simulink model "mass_spring"  (R2017a)
settings: Solver=FixedStepDiscrete  StartTime=0.0  StopTime=inf  RelTol=1e-3  EnableMultiTasking=on
values from neighbouring files (symbols this model uses):
  PWM_Counter_Period = CPU_frequency/PWM_frequency/2    (= 2250)    [pwmset.m]
undefined symbols (not defined in the file or in its folder): DiscIntNeverNeededParam, Down, GPTRIP1SEL, GPTRIP2SEL, TZ1, TZ2, Up
libraries: c2802xlib x2, c280xlib x2, c2806xlib x2, dspsrcs4 x1, dspsigops x1
settings Model: ExtModeTrigDuration=10  Creator=Kalman  LastModifiedBy=ata.otaran
settings DataIOCC: LimitDataPoints=on  SaveFormat=Array
settings OptimizationCC: LifeSpan=Inf  MaxStackSize=512
settings DebuggingCC: AllowSymbolicDim=off  SFUnexpectedBacktrackingDiag=warning  SFNoUnconditionalDefaultTransitionDiag=warning  SFExecutionAtInitializationDiag=none
settings HardwareCC: ProdBitPerChar=16  ProdBitPerInt=16  ProdBitPerPointer=16  ProdBitPerSizeT=32  ProdBitPerPtrDiffT=32  ProdLargestAtomicInteger=Integer  ProdLargestAtomicFloat=None  ProdWordSize=16  ProdLongLongMode=on  ProdHWDeviceType=Texas Instruments->C2000
settings ModelReferenceCC: PropagateSignalLabelsOutOfModel=off
settings SFSimCC: MATLABDynamicMemAlloc=off
settings RTWCC: SystemTargetFile=ert.tlc  HardwareBoard=TI Piccolo F2806x  TLCOptions=-aInlineSetEventsForThisBaseRateFcn=TLC_FALSE -aSuppressMultiTaskScheduler=TLC_FALSE -aRateBasedStepFcn=1  TemplateMakefile=ert_default_tmf  Description=Embedded Coder  Toolchain=Texas Instruments Code Composer Studio v5 (C2000)
settings CodeAppCC: IgnoreCustomStorageClasses=off
settings ERTTargetCC: CodeReplacementLibrary=TI C28x  MultiwordLength=2048  ConvertIfToSwitch=off  SuppressUnreachableDefaultCases=off
settings ConfigComp: CovMetricSettings=dw  CovHtmlReporting=on  CovSaveCumulativeToWorkspaceVar=on  CovSaveSingleToWorkspaceVar=on  CovExternalEMLEnable=off

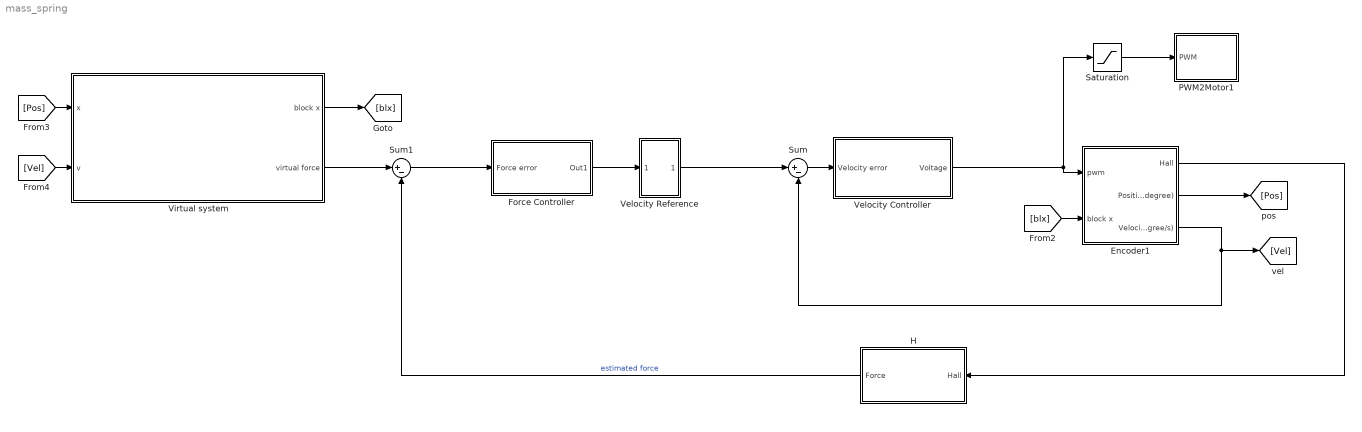
== system mass_spring ==
  Encoder1 : Subsystem
  Force Controller : Subsystem
  H : Subsystem
  PWM2Motor1 : Subsystem
  Saturation : Saturate  UpperLimit=2250  LowerLimit=-2250
  Sum : Sum  Inputs=|+-
  Sum1 : Sum  Inputs=|+-
  Velocity Controller : Subsystem
  Velocity Reference : Subsystem
  Virtual system : Subsystem
  wires:
  Encoder1/2("Position(degree) ") -> [Pos]
  Saturation/1 -> PWM2Motor1/1(PWM)
  Encoder1/3(Velocity(degree/s)) -> Sum/2, [Vel]
  Sum/1 -> Velocity Controller/1("Velocity error ")
  H/1(Force) -> Sum1/2  "estimated force"
  Force Controller/1(Out1) -> Velocity Reference/1(In1)
  Encoder1/1("Hall ") -> H/1(Hall)
  Velocity Reference/1(Out1) -> Sum/1
  Velocity Controller/1(Voltage) -> Saturation/1, Encoder1/1(pwm)
  [blx] -> Encoder1/2(block x)
  Virtual system/1(block x) -> [blx]
  Virtual system/2(virtual force) -> Sum1/1
  Sum1/1 -> Force Controller/1(Force error)
  [Pos] -> Virtual system/1(x)
  [Vel] -> Virtual system/2(v)

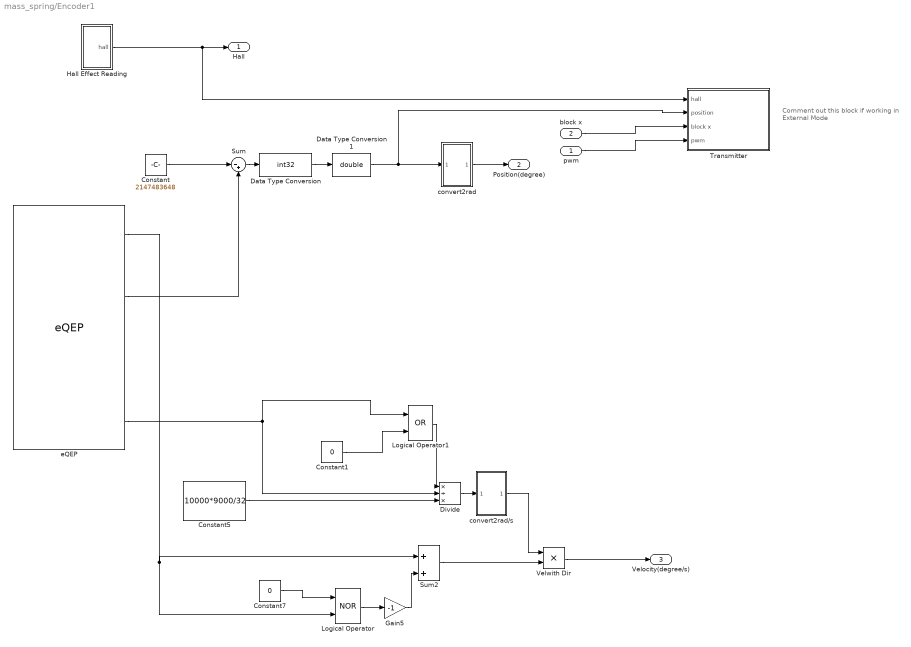
== system mass_spring/Encoder1 ==
  note: Comment out this block if
      | working in External Mode
  pwm : Inport
  block x : Inport  Port=2
  Constant : Constant  Value=2147483648  OutDataTypeStr=uint32
  Constant1 : Constant  Value=0
  Constant5 : Constant  Value=10000*9000/32
  Constant7 : Constant  Value=0
  Data Type Conversion : DataTypeConversion  OutDataTypeStr=int32
  Data Type Conversion1 : DataTypeConversion  OutDataTypeStr=double
  Divide : Product  Inputs=*/*
  Gain5 : Gain  Gain=-1
  Hall Effect Reading : Subsystem
  Logical Operator : Logic  Operator=NOR  AllPortsSameDT=off  OutDataTypeStr=boolean
  Logical Operator1 : Logic  Operator=OR  AllPortsSameDT=off  OutDataTypeStr=boolean
  Sum : Sum  Inputs=|-+
  Sum2 : Sum  Inputs=|++
  Transmitter : Subsystem
  "Velwith Dir " : Product
  convert2rad : Subsystem
  "convert2rad/s " : Subsystem
  eQEP : c280xlib/eQEP  useModule=eQEP1  pcInputmode=Quadrature-count  externalClockrate=2x resolution: Count the rising/falling edge  swapPolarityselection=Clockwise  qdfOutputport=on  qapPolarityselection=off  qbpPolarityselection=off  qipPolarityselection=off  qspPolarityselection=off  igatePolarityselection=off  sampleTime=0.0001  pcOutputport=on  pcMaximumvalue=4294967295  indexInitializationcheck=off  indexInitializationevent=Rising edge  strobeInitializationcheck=off  strobeInitializationevent=Rising edge  softwareInitializationcheck=on  softwareInitializationsource=Set to init value at start up  softwareInitializationmode=on  pcInitialvalue=2147483648  pcResetmode=Reset on an index event  ieloutputport=off  indexEventlatch=Rising edge  seloutputport=off  strobeEventlatch=Rising edge  pcefOutputport=off  enableEqepcapture=on  qctmrOutputport=on  qcprdOutputport=on  captureTimerprescaler=128  upEventprescaler=4  overflowErrorflag=off  directionErrorflag=off  captureTimerposition=On position counter read  unitTimerperiod=1000000000  captureTimerlatch=off  capturePeriodlatch=off  positionCounterlatch=off  soenPolarityselection=off  spselPolarityselection=Index pin is used for sync output  compareValuesource=Specify via dialog  shadowMode=Load on QPOSCNT=0  compareValue=4294967295  syncOutputwidth=1  polaritySyncoutput=Active high  watchdogEnable=off  watchdogTimer=65535  outport1Datatype=auto  outport2Datatype=uint32  outport3Datatype=auto  outport4Datatype=auto  outport5Datatype=auto  outport6Datatype=auto  outport7Datatype=auto  outport8Datatype=auto  outport9Datatype=auto  outport10Datatype=auto  outport11Datatype=auto  outport12Datatype=auto  eqepinterrupt_pce=off  eqepinterrupt_qpe=off  eqepinterrupt_qdc=off  eqepinterrupt_wto=off  eqepinterrupt_pcu=off  eqepinterrupt_pco=off  eqepinterrupt_pcr=off  eqepinterrupt_pcm=off  eqepinterrupt_sel=off  eqepinterrupt_iel=off  eqepinterrupt_uto=off  pheOutputport=off  watchdogOutputport=off  outport13Datatype=auto  outport14Datatype=auto
      settings: SourceProductName=Embedded Coder Support Package for Texas Instruments C2000 Processors  SourceProductBaseCode=TIC2000
  "Hall " : Outport
  "Position(degree) " : Outport  Port=2
  Velocity(degree/s) : Outport  Port=3
  wires:
  "convert2rad/s "/1(Out1) -> "Velwith Dir "/1
  Hall Effect Reading/1(hall) -> Transmitter/1(hall), "Hall "/1
  Logical Operator1/1 -> Divide/1
  Constant5/1 -> Divide/3
  Constant1/1 -> Logical Operator1/2
  Sum2/1 -> "Velwith Dir "/2
  Constant7/1 -> Logical Operator/1
  Logical Operator/1 -> Gain5/1
  Divide/1 -> "convert2rad/s "/1(In1)
  Gain5/1 -> Sum2/2
  eQEP/1 -> Logical Operator/2, Sum2/1
  eQEP/2 -> Sum/2
  Constant/1 -> Sum/1
  eQEP/4 -> Divide/2, Logical Operator1/1
  "Velwith Dir "/1 -> Velocity(degree/s)/1
  Data Type Conversion/1 -> Data Type Conversion1/1
  convert2rad/1(Out1) -> "Position(degree) "/1
  Sum/1 -> Data Type Conversion/1
  Data Type Conversion1/1 -> Transmitter/2(position), convert2rad/1(In1)
  pwm/1 -> Transmitter/4(pwm)
  block x/1 -> Transmitter/3(block x)

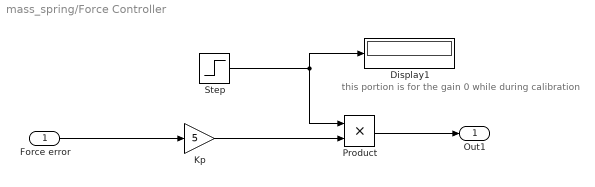
== system mass_spring/Force Controller ==
  note: this portion is for the gain 0 while during calibration
  Force error : Inport
  Display1 : Display
  Kp : Gain  Gain=5
  Product : Product
  Step : Step  Time=0.2
  Out1 : Outport
  wires:
  Force error/1 -> Kp/1
  Product/1 -> Out1/1
  Kp/1 -> Product/2
  Step/1 -> Product/1, Display1/1

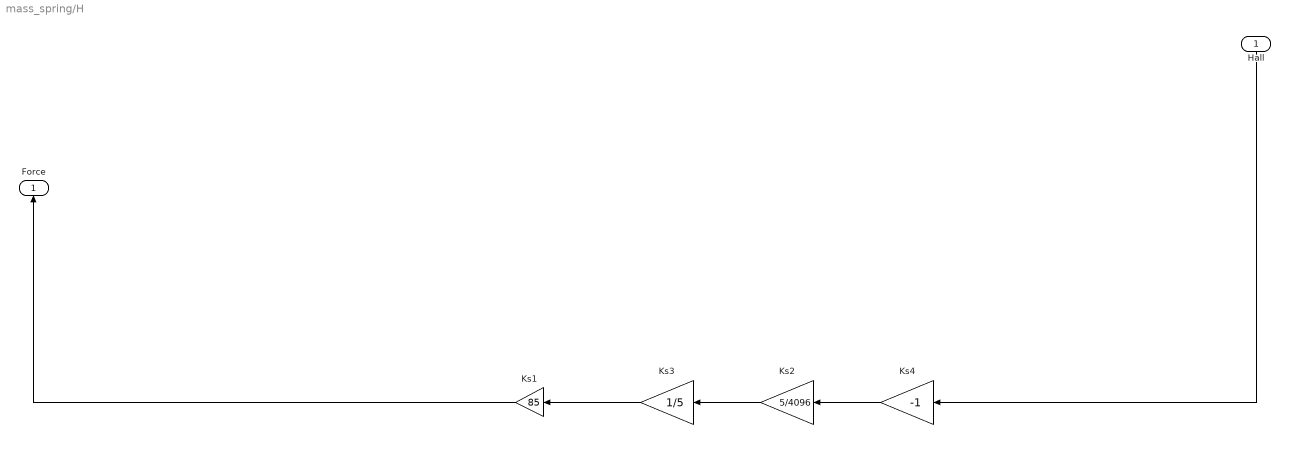
== system mass_spring/H ==
  Hall : Inport
  Ks1 : Gain  Gain=85
  Ks2 : Gain  Gain=5/4096
  Ks3 : Gain  Gain=1/5
  Ks4 : Gain  Gain=-1
  Force : Outport
  wires:
  Hall/1 -> Ks4/1
  Ks1/1 -> Force/1
  Ks4/1 -> Ks2/1
  Ks2/1 -> Ks3/1
  Ks3/1 -> Ks1/1

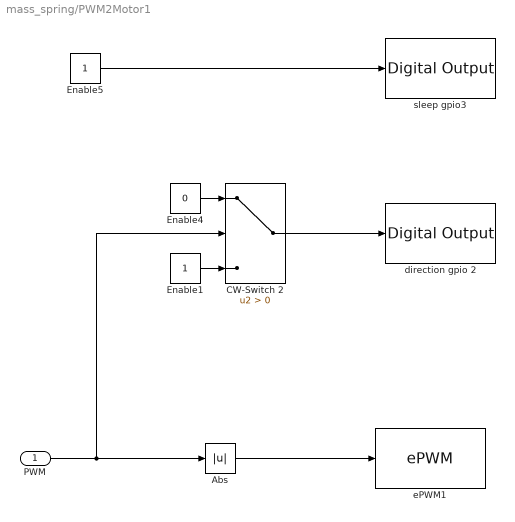
== system mass_spring/PWM2Motor1 ==
  PWM : Inport
  Abs : Abs
  CW-Switch 2 : Switch  Criteria=u2 > Threshold
  Enable1 : Constant
  Enable4 : Constant  Value=0
  Enable5 : Constant
  direction gpio 2 : c2806xlib/Digital Output  GPIO_Number=GPIO0~GPIO7  GPIO_Bit0=off  GPIO_BIT0_Toggle=off  GPIO_Bit1=off  GPIO_BIT1_Toggle=off  GPIO_Bit2=on  GPIO_BIT2_Toggle=off  GPIO_Bit3=off  GPIO_BIT3_Toggle=off  GPIO_Bit4=off  GPIO_BIT4_Toggle=off  GPIO_Bit5=off  GPIO_BIT5_Toggle=off  GPIO_Bit6=off  GPIO_BIT6_Toggle=off  GPIO_Bit7=off  GPIO_BIT7_Toggle=off
      settings: SourceProductName=Embedded Coder Support Package for Texas Instruments C2000 Processors  SourceProductBaseCode=TIC2000
  ePWM1 : c2802xlib/ePWM  useModule=ePWM1  ePWMxLINKTBPRD=Not Linked  periodUnits=Clock cycles  timerSource=Specify via dialog  timerPeriod_clk=PWM_Counter_Period+1  timerPeriod_sec=0.0001  tbshadow=Counter equals to zero  countingMode=Up-Down  phaseActiveEnable=Disable  phaseDirection=Count down after sync  phaseActive=0  synchronizationEnable=off  dcaevt1Sync=off  dcbevt1Sync=off  synchronizationOption=Disable  clockPrescale=1  HSclockPrescale=1  enswap=off  ePWMxAStatus=on  ePWMxAactionLogic1=Do nothing  ePWMxAactionLogic2=Do nothing  ePWMxAactionLogic3=Clear  ePWMxAactionLogic4=Set  ePWMxAactionLogic5=Do nothing  ePWMxAactionLogic6=Do nothing  ePWMxALoadMode=Load on counter equals to zero (CTR=Zero)  ePWMxACSFenable=off  ePWMxACSFvalue=Forcing disable  ePWMxASFreload=Zero  ePWMxBStatus=off  ePWMxBactionLogic1=Set  ePWMxBactionLogic2=Clear  ePWMxBactionLogic3=Do nothing  ePWMxBactionLogic4=Do nothing  ePWMxBactionLogic5=Clear  ePWMxBactionLogic6=Set  ePWMxBLoadMode=Load on counter equals to zero (CTR=Zero)  ePWMxBCSFenable=off  ePWMxBCSFvalue=Forcing disable  ePWMxBSFreload=Zero  ePWNxBOutWay=off  ePWMxLINKCMPA=Not Linked  CMPAUnits=Clock cycles  CMPASource=Input port  CMPAValue_per=50  CMPAValue_clk=PWM_Counter_Period/2+1  enCMPAshadow=Counter equals to zero  ePWMxLINKCMPB=Not Linked  CMPBUnits=Clock cycles  CMPBSource=Specify via dialog  CMPBValue_per=50  CMPBValue_clk=PWM_Counter_Period/2+1  enCMPBshadow=Counter equals to zero  ePWMxLINKCMPC=Not Linked  CMPCUnits=Clock cycles  CMPCSource=Specify via dialog  CMPCValue_per=50  CMPCValue_clk=32000  enCMPCshadow=Counter equals to zero  ePWMxLINKCMPD=Not Linked  CMPDUnits=Clock cycles  CMPDSource=Specify via dialog  CMPDValue_per=50  CMPDValue_clk=32000  enCMPDshadow=Counter equals to zero  enableDBePWMxA=off  enableDBePWMxB=off  enhalfcycle=off  DBpolarity=Active high (AH)  DBedgeDelay=Positive  DBSource_ePWMxA=ePWMxA  DBSource_ePWMxB=ePWMxA  DBperiodSource=Specify via dialog  REDperiod=0  FEDperiod=0  adcstartModuleA=off  adcrequestEventA=First event  adcstartEventA=Digital Compare Module A Event 1 start of conversion (DCAEVT1.soc)  adcstartEventA_type2=Digital Compare Module A Event 1 start of conversion (DCAEVT1.soc)  adcstartModuleB=off  adcrequestEventB=First event  adcstartEventB=Counter equals to zero (CTR=Zero)  adcstartEventB_type2=Counter equals to zero (CTR=Zero)  intEn=off  intPrd=First event  intSel=Counter equals to zero (CTR=Zero)  intSel_type2=Counter equals to zero (CTR=Zero)  hrpe=off  enHRPWM=off  HRPWM_LoadMode=Counter equals to period (CTR=PRD)  HRPWM_CTLMode=Duty or Period control mode  HRPWM_EDGMode=Both edge  hrpeb=off  enHRPWMB=off  HRPWM_LoadModeB=Counter equals to zero (CTR=ZERO)  HRPWM_CTLModeB=Duty or Period control mode  HRPWM_EDGModeB=Both edge  enSFO=on  enautoconv=on  chopperEnable=off  chopperFrequency=1  chopperFirstwidth=1  chopperDuty=12.5%  tripZonesource=Specify via dialog  tzselOSHT1=off  tzselOSHT2=off  tzselOSHT3=off  tzselOSHDCAEV1=off  tzselOSHDCBEV1=off  tzselCBC1=off  tzselCBC2=off  tzselCBC3=off  tzselCBCDCAEV2=off  tzselCBCDCBEV2=off  tzselOSHT4=off  tzselOSHT5=off  tzselOSHT6=off  tzselCBC4=off  tzselCBC5=off  tzselCBC6=off  enTzOstIntr=off  enTzCbcIntr=off  enTzDCAEVT1Intr=off  enTzDCAEVT2Intr=off  enTzDCBEVT1Intr=off  enTzDCBEVT2Intr=off  ePWMxAforced=No action  ePWMxBforced=No action  DCAEVT1forced=No action  DCBEVT1forced=No action  DCAEVT2forced=No action  DCBEVT2forced=No action  dcah=Trip Zone 1 input (TZ1)  dcal=Trip Zone 2 input (TZ2)  dcbh=Trip Zone 1 input (TZ1)  dcbl=Trip Zone 2 input (TZ2)  dcah_type2=GPTRIP1SEL/(TZ1)  dcal_type2=GPTRIP2SEL/(TZ2)  dcbh_type2=GPTRIP1SEL/(TZ1)  dcbl_type2=GPTRIP2SEL/(TZ2)  gendcaevt1=Event disabled  gendcaevt2=Event disabled  gendcbevt1=Event disabled  gendcbevt2=Event disabled  dcaevt1src=DCAEVT1 with sync  dcaevt2src=DCAEVT2 with sync  dcbevt1src=DCBEVT1 with sync  dcbevt2src=DCBEVT2 with sync  pulsesel=Counter equals to zero (CTR=Zero)  blankinv=off  blankoffset=0  blankwidth=0  evsrcsel=Filtered version of DCAEVT1 (DCAEVT1FILT)  encape=off  PwmType=C2000
      settings: SourceProductName=Embedded Coder Support Package for Texas Instruments C2000 Processors
  sleep gpio3 : c2806xlib/Digital Output  GPIO_Number=GPIO0~GPIO7  GPIO_Bit0=off  GPIO_BIT0_Toggle=off  GPIO_Bit1=off  GPIO_BIT1_Toggle=off  GPIO_Bit2=off  GPIO_BIT2_Toggle=off  GPIO_Bit3=on  GPIO_BIT3_Toggle=off  GPIO_Bit4=off  GPIO_BIT4_Toggle=off  GPIO_Bit5=off  GPIO_BIT5_Toggle=off  GPIO_Bit6=off  GPIO_BIT6_Toggle=off  GPIO_Bit7=off  GPIO_BIT7_Toggle=off
      settings: SourceProductName=Embedded Coder Support Package for Texas Instruments C2000 Processors  SourceProductBaseCode=TIC2000
  wires:
  PWM/1 -> Abs/1, CW-Switch 2/2
  Enable1/1 -> CW-Switch 2/3
  Enable4/1 -> CW-Switch 2/1
  Enable5/1 -> sleep gpio3/1
  CW-Switch 2/1 -> direction gpio 2/1
  Abs/1 -> ePWM1/1

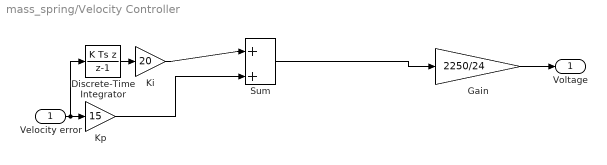
== system mass_spring/Velocity Controller ==
  "Velocity error " : Inport
  Discrete-Time Integrator : DiscreteIntegrator  IntegratorMethod=Integration: Backward Euler  InitialConditionSetting=State (most efficient)  SampleTime=-1  ICPrevOutput=DiscIntNeverNeededParam  ICPrevScaledInput=DiscIntNeverNeededParam
  Gain : Gain  Gain=2250/24
  Ki : Gain  Gain=20
  Kp : Gain  Gain=15
  Sum : Sum  Inputs=|++
  Voltage : Outport
  wires:
  "Velocity error "/1 -> Discrete-Time Integrator/1, Kp/1
  Kp/1 -> Sum/2
  Ki/1 -> Sum/1
  Sum/1 -> Gain/1
  Discrete-Time Integrator/1 -> Ki/1
  Gain/1 -> Voltage/1

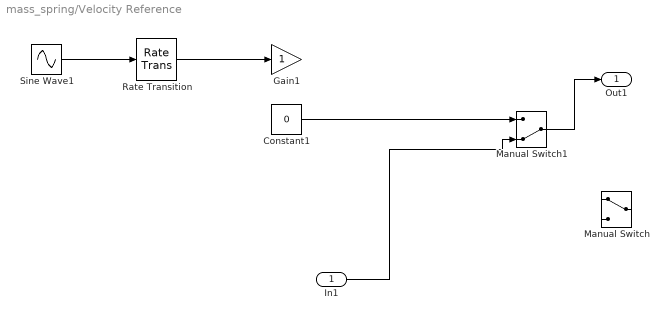
== system mass_spring/Velocity Reference ==
  In1 : Inport
  Constant1 : Constant  Value=0
  Gain1 : Gain
  Manual Switch : ManualSwitch
  Manual Switch1 : ManualSwitch  CurrentSetting=0
  Rate Transition : RateTransition
  Sine Wave1 : Sin  Amplitude=pi  Frequency=2*pi  SampleTime=1e-3
  Out1 : Outport
  wires:
  In1/1 -> Manual Switch1/2
  Rate Transition/1 -> Gain1/1
  Constant1/1 -> Manual Switch1/1
  Sine Wave1/1 -> Rate Transition/1
  Manual Switch1/1 -> Out1/1

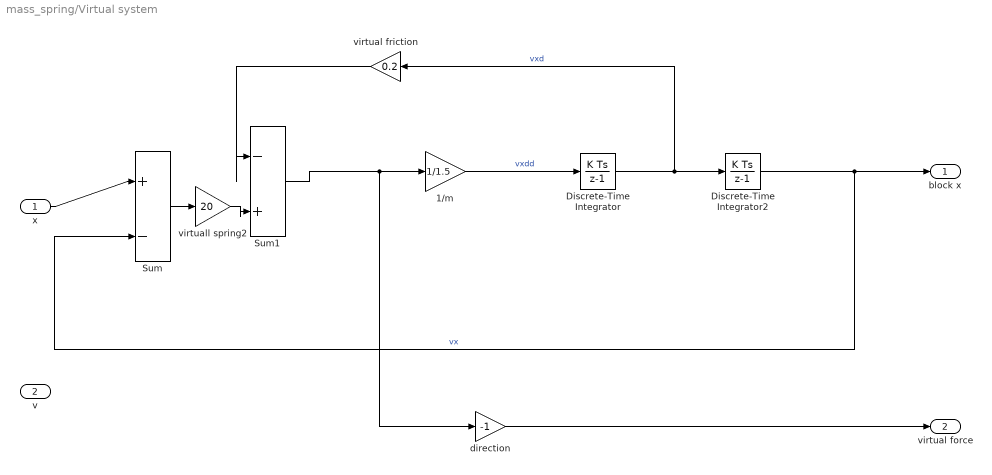
== system mass_spring/Virtual system ==
  x : Inport
  v : Inport  Port=2
  " virtual friction" : Gain  Gain=0.2
  1/m : Gain  Gain=1/1.5
  Discrete-Time Integrator : DiscreteIntegrator  InitialConditionSetting=State (most efficient)  SampleTime=-1  ICPrevOutput=DiscIntNeverNeededParam  ICPrevScaledInput=DiscIntNeverNeededParam
  Discrete-Time Integrator2 : DiscreteIntegrator  InitialConditionSetting=State (most efficient)  SampleTime=-1  ICPrevOutput=DiscIntNeverNeededParam  ICPrevScaledInput=DiscIntNeverNeededParam
  Sum : Sum  Inputs=|+-
  Sum1 : Sum  Inputs=|-+
  direction : Gain  Gain=-1
  virtuall spring2 : Gain  Gain=20
  block x : Outport
  virtual force : Outport  Port=2
  wires:
  Discrete-Time Integrator/1 -> " virtual friction"/1, Discrete-Time Integrator2/1  "vxd"
  Discrete-Time Integrator2/1 -> block x/1, Sum/2  "vx"
  Sum1/1 -> 1/m/1, direction/1
  x/1 -> Sum/1
  1/m/1 -> Discrete-Time Integrator/1  "vxdd"
  Sum/1 -> virtuall spring2/1
  virtuall spring2/1 -> Sum1/2
  " virtual friction"/1 -> Sum1/1
  direction/1 -> virtual force/1

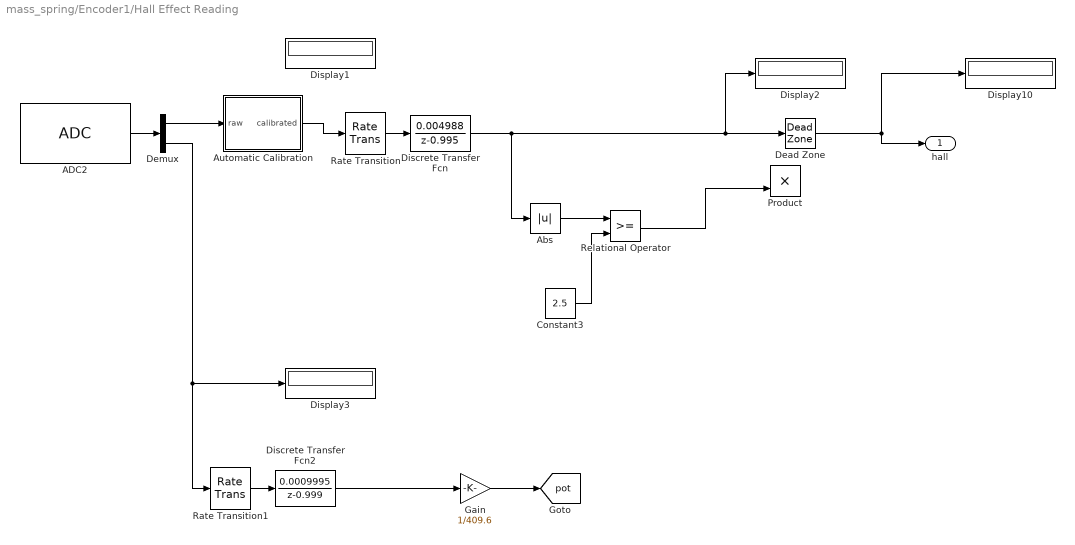
== system mass_spring/Encoder1/Hall Effect Reading ==
  ADC2 : c2802xlib/ADC  ADCModule=1  samplingMode=Simultaneous sample mode  ADCResolution=12-bit (Single-ended input)  useSOC1=SOC1  useSOC2=SOC0_SOC1  SOCAcquisitionWindow=7  SOCTriggerSource=Software  SOCInterruptTrigger=No ADCINT  Ts=-1  dType=int32  postInterrupt=off  interruptSel=ADCINT1  ADCINTContinuous=off  endma=off  chdma=1  blkParamProc=C2000  conv1=ADCINA7  conv2=ADCINA7 and ADCINB7  conv1_Type4=ADCIN0  conv2_Type4=ADCIN0 and ADCIN1
      settings: SourceProductName=Embedded Coder Support Package for Texas Instruments C2000 Processors
  Abs : Abs
  Automatic Calibration : Subsystem
  Constant3 : Constant  Value=2.5
  Dead Zone : DeadZone  LowerValue=-2.5  UpperValue=2.5  SaturateOnIntegerOverflow=on
  Demux : Demux  Outputs=2
  Discrete Transfer Fcn : DiscreteTransferFcn  Numerator=[0.004988]  Denominator=[1 -0.995]
  Discrete Transfer Fcn2 : DiscreteTransferFcn  Numerator=[0.0009995]  Denominator=[1 -0.999]
  Display{1..3,10} (4 alike) : Display
  Gain : Gain  Gain=1/409.6  OutDataTypeStr=double
  Product : Product
  Rate Transition : RateTransition
  Rate Transition1 : RateTransition
  Relational Operator : RelationalOperator  OutDataTypeStr=boolean  RndMeth=Nearest
  hall : Outport
  tag scope: pot=global
  wires:
  Abs/1 -> Relational Operator/1
  Constant3/1 -> Relational Operator/2
  Relational Operator/1 -> Product/2
  Automatic Calibration/1(calibrated) -> Rate Transition/1
  Rate Transition/1 -> Discrete Transfer Fcn/1
  ADC2/1 -> Demux/1
  Demux/2 -> Display3/1, Rate Transition1/1
  Rate Transition1/1 -> Discrete Transfer Fcn2/1
  Discrete Transfer Fcn2/1 -> Gain/1
  Discrete Transfer Fcn/1 -> Abs/1, Dead Zone/1, Display2/1
  Gain/1 -> [pot]
  Dead Zone/1 -> hall/1, Display10/1
  Demux/1 -> Automatic Calibration/1(raw)

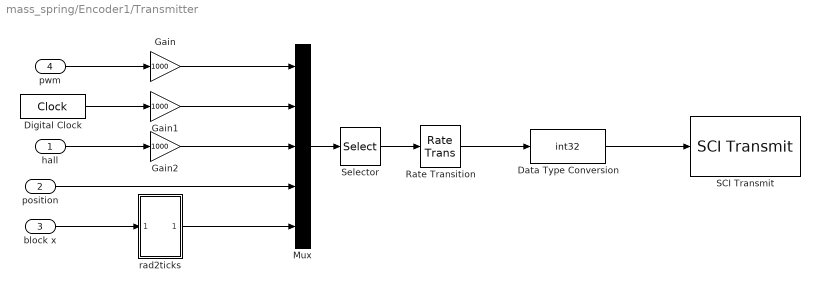
== system mass_spring/Encoder1/Transmitter ==
  hall : Inport
  position : Inport  Port=2
  block x : Inport  Port=3
  pwm : Inport  Port=4
  Data Type Conversion : DataTypeConversion  OutDataTypeStr=int32  ConvertRealWorld=Stored Integer (SI)
  Digital Clock : DigitalClock  SampleTime=0.0001
  Gain : Gain  Gain=1000
  Gain1 : Gain  Gain=1000
  Gain2 : Gain  Gain=1000
  Mux : Mux  Inputs=5
  Rate Transition : RateTransition  Integrity=off  OutPortSampleTime=0.01
  SCI Transmit : c280xlib/SCI Transmit  sciModule=A  dataHead='S'  dataTail='E'  postInterrupt=on  numFifo=3
      settings: SourceProductName=Embedded Coder Support Package for Texas Instruments C2000 Processors
  Selector : Selector  InputPortWidth=5  IndexOptions=Index vector (dialog)  Indices=[4 5]  OutputSizes=1
  rad2ticks : Subsystem
  wires:
  rad2ticks/1(Out1) -> Mux/5
  position/1 -> Mux/4
  Rate Transition/1 -> Data Type Conversion/1
  Data Type Conversion/1 -> SCI Transmit/1
  block x/1 -> rad2ticks/1(In1)
  Digital Clock/1 -> Gain1/1
  Gain/1 -> Mux/1
  pwm/1 -> Gain/1
  hall/1 -> Gain2/1
  Mux/1 -> Selector/1
  Gain1/1 -> Mux/2
  Gain2/1 -> Mux/3
  Selector/1 -> Rate Transition/1

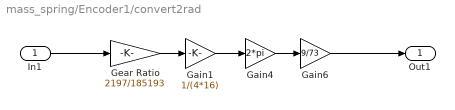
== system mass_spring/Encoder1/convert2rad ==
  In1 : Inport
  Gain1 : Gain  Gain=1/(4*16)
  Gain4 : Gain  Gain=2*pi
  Gain6 : Gain  Gain=9/73
  Gear Ratio : Gain  Gain=2197/185193
  Out1 : Outport
  wires:
  Gain1/1 -> Gain4/1
  Gear Ratio/1 -> Gain1/1
  Gain4/1 -> Gain6/1
  In1/1 -> Gear Ratio/1
  Gain6/1 -> Out1/1

== system mass_spring/Encoder1/convert2rad//s  ==
  In1 : Inport
  Gain1 : Gain  Gain=1/(4*16)
  Gain4 : Gain  Gain=2*pi
  Gain6 : Gain  Gain=9/73
  Gear Ratio : Gain  Gain=2197/185193
  Out1 : Outport
  wires:
  Gain6/1 -> Out1/1
  In1/1 -> Gear Ratio/1
  Gain4/1 -> Gain6/1
  Gear Ratio/1 -> Gain1/1
  Gain1/1 -> Gain4/1

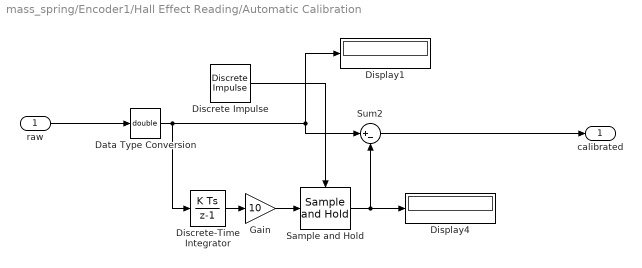
== system mass_spring/Encoder1/Hall Effect Reading/Automatic Calibration ==
  raw : Inport
  Data Type Conversion : DataTypeConversion  OutDataTypeStr=double
  Discrete Impulse : dspsrcs4/Discrete  Impulse  Delay=1000  SampleTime=-1  FrameSample=1  OutputFrames=off  dataType=double  isSigned=on  wordLen=16  udDataType=sfix(16)  fracBitsMode=Best precision  numFracBits=15  OutDataTypeStr=double  LastOutDataTypeStr=double
  Discrete-Time Integrator : DiscreteIntegrator  InitialConditionSetting=State (most efficient)  SampleTime=0.0001  ICPrevOutput=DiscIntNeverNeededParam  ICPrevScaledInput=DiscIntNeverNeededParam
  Display1 : Display
  Display4 : Display
  Gain : Gain  Gain=10
  Sample and Hold : dspsigops/Sample and Hold  trig=Rising edge  initCond=0  latchinput=off
  Sum2 : Sum  Inputs=|+-
  calibrated : Outport
  wires:
  raw/1 -> Data Type Conversion/1
  Discrete Impulse/1 -> Sample and Hold/Trigger
  Data Type Conversion/1 -> Discrete-Time Integrator/1, Sum2/1, Display1/1
  Sample and Hold/1 -> Display4/1, Sum2/2
  Discrete-Time Integrator/1 -> Gain/1
  Gain/1 -> Sample and Hold/1
  Sum2/1 -> calibrated/1

== system mass_spring/Encoder1/Transmitter/rad2ticks ==
  In1 : Inport
  Gain1 : Gain  Gain=4*16
  Gain4 : Gain  Gain=1/(2*pi)
  Gain6 : Gain  Gain=73/9
  Gear Ratio : Gain  Gain=185193/2197
  Out1 : Outport
  wires:
  Gain1/1 -> Gain4/1
  Gear Ratio/1 -> Gain1/1
  Gain4/1 -> Gain6/1
  In1/1 -> Gear Ratio/1
  Gain6/1 -> Out1/1
